simulink model "tqdtqr_rebuild_V3"  (R2021b)
settings: Solver=VariableStepAuto  StartTime=0.0  StopTime=10.0  RelTol=1e-3
undefined symbols (not defined in the file): ATQD_AfterTqMinGain_X_Deg, ATQD_APSCreepBaseTqD_X_kph, ATQD_APSCreepBaseTqD_Y_Deg, ATQD_APSCreepBaseTqR_X_kph, ATQD_APSCreepBaseTqR_Y_Deg, ATQD_APSCreepIterm_X_kph, ATQD_APSCreepIterm_Y_kph, ATQD_APSCreepPterm_X_kph, ATQD_APSCreepPterm_Y_kph, ATQD_APSDecReq_X_kph, ATQD_APSDecReq_Y_mps2, ATQD_APSDecReqCMD_X_kph, ATQD_APSDecReqTs_X_pct, ATQD_APSDecTimeGain_X_Deg, ATQD_APSDecTimeGain_Y_s, ATQD_APSReqLowSpd_X_Deg, ATQD_AutoHoldReleaseBPS_X_Deg, ATQD_AWDLoadTrqnsGain_X_kg, ATQD_AWDLoadTrqnsGain_Y_pct, ATQD_BOSEnBPSPosn_X_kph, ATQD_BOSMap_X_rpm, ATQD_BOSMap_Y_pct, ATQD_CreepBaseTqD_X_kph, ATQD_CreepBaseTqD_Y_Deg, ATQD_CreepBaseTqR_X_kph, ATQD_CreepBaseTqR_Y_Deg, ATQD_CreepBPSDisPosn_X_Deg, ATQD_CreepBPSDisPosnR_X_Deg, ATQD_CreepBPSEnPosn_X_Deg, ATQD_CreepBPSEnPosnR_X_Deg, ATQD_CreepDeltaTq_X_kph, ATQD_CreepIterm_X_kph, ATQD_CreepIterm_Y_kph, ATQD_CreepItermMaxLimit_X_pct, ATQD_CreepPreloadTime_X_kph, ATQD_CreepPreloadTq_X_kph, ATQD_CreepPreloadTq_Y_s, ATQD_CreepProtTq_X_Deg, ATQD_CreepPterm_X_kph, ATQD_CreepPterm_Y_kph, ATQD_CreepRrTqSpRat_X_rpm, ATQD_CreepRrTqSpRat_Y_Nm, ATQD_CreepTargetSpdD_X_pct, ATQD_CreepTargetSpdR_X_pct, ATQD_CreepUpLimitTq_X_rpm, ATQD_DecIneOPDHoldEnDelay_X_Deg, ATQD_DecIneOPDHoldEnDelay_Y_bar, ATQD_ECOTqMapD_X_rpm, ATQD_ECOTqMapD_Y_pct, ATQD_EMTqMapD_X_rpm, ATQD_EMTqMapD_Y_pct, ATQD_EOPDTqMapDCon_X_rpm, ATQD_EOPDTqMapDCon_Y_Deg, ATQD_EstInitVehWeight_X_c, ATQD_FAfterTqCMDGain_X_rpm, ATQD_FAfterTqCMDGain_Y_pct, ATQD_ForceLowSpd_X_Deg, ATQD_ForcePLimitSpd_X_Deg, ATQD_FrLossMAPLowV_X_rpm, ATQD_FrLossMAPLowV_Y_Nm ... (+949)
libraries: simulink x235, hcu_lib x208, tqr x63, tqd x6
(part 31 of 37)

== system tqdtqr_rebuild_V3/Input_Convert/Signal function/combo key/Combo Key Detection/DiagnosisOff Mode/Key1 ==
  VSCP_ComboKeyCMD_enum : Inport
  VSCP_ComboKeyEn_flg : Inport  Port=2
  VSCP_ComboKeyReset_flg : Inport  Port=3
  AND : Logic  Inputs=3  AllPortsSameDT=off  OutDataTypeStr=boolean
  Constant1 : Constant  Value=KTQD_DiagnosisOff1_enum
  Constant2 : Constant  Value=ENUM_COMBOKEY_NONE
  Constant4 : Constant  Value=ENUM_COMBOKEY_NONE
  Data Type Conversion : DataTypeConversion  OutDataTypeStr=uint8
  Delay : Delay  DelayLength=1  InitialCondition=uint8(0)
      settings: AttributesFormatString=%<InitialCondition>
  Delay1 : Delay  DelayLength=1  InitialCondition=uint8(0)
      settings: AttributesFormatString=%<InitialCondition>
  Detect Change : simulink/Logic and Bit Operations/Detect Change  vinit=boolean(0)  OutDataTypeStr=boolean
  Detect Increase : simulink/Logic and Bit Operations/Detect Increase  vinit=boolean(0)  OutDataTypeStr=boolean
  Equal : RelationalOperator  Operator===  OutDataTypeStr=boolean  RndMeth=Simplest
  Equal1 : RelationalOperator  Operator=~=  OutDataTypeStr=boolean  RndMeth=Simplest
  Equal2 : RelationalOperator  Operator===  OutDataTypeStr=boolean  RndMeth=Simplest
  If : If  NumInputs=2  IfExpression=u1 ~=0  ElseIfExpressions=u2 ~= 0
  Maintain : Subsystem  TreatAsAtomicUnit=on
  Merge : Merge  Inputs=3
  OR : Logic  Operator=OR  AllPortsSameDT=off  OutDataTypeStr=boolean
  Reset : Subsystem  TreatAsAtomicUnit=on
  Write : Subsystem  TreatAsAtomicUnit=on
  VSCP_ComboKey1_enum : Outport
  VSCP_Key1Pass_flg : Outport  Port=2
  wires:
  OR/1 -> [VSCP_ResetComboKey_flg]  "VSCP_ResetComboKey_flg"
  [VSCP_WriteComboCMD_flg] -> If/2
  [VSCP_ComboKeyCMD_enum] -> Equal1/1
  [VSCP_ComboKeyReset_flg] -> OR/2
  [VSCP_ComboKey1_enum] -> Delay/1
  Equal1/1 -> AND/2
  Constant2/1 -> Equal2/2
  Equal2/1 -> AND/3
  Reset/1(ResetToZero) -> Merge/1
  Merge/1 -> Data Type Conversion/1
  Delay/1 -> Equal2/1
  If/3 -> Maintain/Action
  Constant4/1 -> Equal1/2
  Maintain/1(KeepKey1) -> Merge/3
  Detect Change/1 -> AND/1
  [VSCP_ComboKeyEn_flg] -> Detect Increase/1
  [VSCP_ResetComboKey_flg] -> If/1
  [VSCP_ComboKeyCMD_enum] -> Detect Change/1
  [VSCP_ComboKeyCMD_enum] -> Write/1(Input)
  AND/1 -> [VSCP_WriteComboCMD_flg]  "VSCP_WriteComboCMD_flg"
  Detect Increase/1 -> OR/1
  If/1 -> Reset/Action
  Write/1(WriteCMD) -> Merge/2
  If/2 -> Write/Action
  [VSCP_ComboKey1_enum] -> Equal/1
  Constant1/1 -> Equal/2
  Equal/1 -> [VSCP_Key1Pass_flg]  "VTQD_DiagnosisOff1Pass_flg"
  VSCP_ComboKeyCMD_enum/1 -> [VSCP_ComboKeyCMD_enum]
  VSCP_ComboKeyReset_flg/1 -> [VSCP_ComboKeyReset_flg]
  VSCP_ComboKeyEn_flg/1 -> [VSCP_ComboKeyEn_flg]
  [VSCP_ComboKey1_enum] -> VSCP_ComboKey1_enum/1
  [VSCP_Key1Pass_flg] -> VSCP_Key1Pass_flg/1
  [VSCP_ComboKey1_enum] -> Delay1/1
  Delay1/1 -> Maintain/1(Input)
  Data Type Conversion/1 -> [VSCP_ComboKey1_enum]  "VTQD_DiagnosisOff1_enum"

== system tqdtqr_rebuild_V3/Input_Convert/Signal function/combo key/Combo Key Detection/DiagnosisOff Mode/Key2 ==
  VSCP_ComboKeyCMD_enum : Inport
  VSCP_ComboKeyEn_flg : Inport  Port=2
  VSCP_ComboKeyReset_flg : Inport  Port=3
  VSCP_ComboKey1_enum : Inport  Port=4
  AND : Logic  Inputs=4  AllPortsSameDT=off  OutDataTypeStr=boolean
  Constant1 : Constant  Value=KTQD_DiagnosisOff2_enum
  Constant2 : Constant  Value=ENUM_COMBOKEY_NONE
  Constant3 : Constant  Value=ENUM_COMBOKEY_NONE
  Constant4 : Constant  Value=ENUM_COMBOKEY_NONE  OutDataTypeStr=uint8
  Data Type Conversion : DataTypeConversion  OutDataTypeStr=uint8
  Delay : Delay  DelayLength=1  InitialCondition=uint8(0)
      settings: AttributesFormatString=%<InitialCondition>
  Delay1 : Delay  DelayLength=1  InitialCondition=uint8(0)
      settings: AttributesFormatString=%<InitialCondition>
  Delay2 : Delay  DelayLength=1  InitialCondition=uint8(0)
      settings: AttributesFormatString=%<InitialCondition>
  Detect Change : simulink/Logic and Bit Operations/Detect Change  vinit=boolean(0)  OutDataTypeStr=boolean
  Detect Increase : simulink/Logic and Bit Operations/Detect Increase  vinit=boolean(0)  OutDataTypeStr=boolean
  Equal : RelationalOperator  Operator===  OutDataTypeStr=boolean  RndMeth=Simplest
  Equal1 : RelationalOperator  Operator=~=  OutDataTypeStr=boolean  RndMeth=Simplest
  Equal2 : RelationalOperator  Operator=~=  OutDataTypeStr=boolean  RndMeth=Simplest
  Equal3 : RelationalOperator  Operator===  OutDataTypeStr=boolean  RndMeth=Simplest
  If : If  NumInputs=2  IfExpression=u1 ~=0  ElseIfExpressions=u2 ~= 0
  Maintain : Subsystem  TreatAsAtomicUnit=on
  Merge : Merge  Inputs=3
  OR : Logic  Operator=OR  AllPortsSameDT=off  OutDataTypeStr=boolean
  Reset : Subsystem  TreatAsAtomicUnit=on
  Write : Subsystem  TreatAsAtomicUnit=on
  VSCP_ComboKey2_enum : Outport
  VSCP_Key2Pass_flg : Outport  Port=2
  wires:
  [VSCP_Key2Pass_flg] -> VSCP_Key2Pass_flg/1
  [VSCP_ComboKey2_enum] -> VSCP_ComboKey2_enum/1
  VSCP_ComboKeyEn_flg/1 -> [VSCP_ComboKeyEn_flg]
  VSCP_ComboKeyReset_flg/1 -> [VSCP_ComboKeyReset_flg]
  VSCP_ComboKeyCMD_enum/1 -> [VSCP_ComboKeyCMD_enum]
  Equal/1 -> [VSCP_Key2Pass_flg]  "VTQD_DiagnosisOff2Pass_flg"
  Constant1/1 -> Equal/2
  [VSCP_ComboKey2_enum] -> Equal/1
  If/2 -> Write/Action
  Write/1(WriteCMD) -> Merge/2
  If/1 -> Reset/Action
  Detect Increase/1 -> OR/1
  AND/1 -> [VSCP_WriteComboCMD_flg]  "VSCP_WriteComboCMD_flg"
  [VSCP_ComboKeyCMD_enum] -> Write/1(Input)
  [VSCP_ComboKeyCMD_enum] -> Detect Change/1
  [VSCP_ResetComboKey_flg] -> If/1
  [VSCP_ComboKeyEn_flg] -> Detect Increase/1
  Detect Change/1 -> AND/1
  Maintain/1(KeepKey2) -> Merge/3
  Constant4/1 -> Equal1/2
  If/3 -> Maintain/Action
  Delay1/1 -> Equal2/1
  Merge/1 -> Data Type Conversion/1
  Reset/1(ResetToZero) -> Merge/1
  Equal2/1 -> AND/3
  Constant2/1 -> Equal2/2
  Equal1/1 -> AND/2
  [VSCP_ComboKey1_enum] -> Delay1/1
  [VSCP_ComboKeyReset_flg] -> OR/2
  [VSCP_ComboKeyCMD_enum] -> Equal1/1
  [VSCP_WriteComboCMD_flg] -> If/2
  OR/1 -> [VSCP_ResetComboKey_flg]  "VSCP_ResetComboKey_flg"
  VSCP_ComboKey1_enum/1 -> [VSCP_ComboKey1_enum]
  [VSCP_ComboKey2_enum] -> Delay/1
  Constant3/1 -> Equal3/2
  Delay/1 -> Equal3/1
  Equal3/1 -> AND/4
  Delay2/1 -> Maintain/1(Input)
  [VSCP_ComboKey2_enum] -> Delay2/1
  Data Type Conversion/1 -> [VSCP_ComboKey2_enum]  "VTQD_DiagnosisOff2_enum"

== system tqdtqr_rebuild_V3/Input_Convert/Signal function/combo key/Combo Key Detection/DiagnosisOff Mode/Key3 ==
  VSCP_ComboKeyCMD_enum : Inport
  VSCP_ComboKeyEn_flg : Inport  Port=2
  VSCP_ComboKeyReset_flg : Inport  Port=3
  VSCP_ComboKey2_enum : Inport  Port=4
  AND : Logic  Inputs=4  AllPortsSameDT=off  OutDataTypeStr=boolean
  Constant1 : Constant  Value=KTQD_DiagnosisOff3_enum
  Constant2 : Constant  Value=ENUM_COMBOKEY_NONE
  Constant3 : Constant  Value=ENUM_COMBOKEY_NONE
  Constant4 : Constant  Value=ENUM_COMBOKEY_NONE
  Data Type Conversion : DataTypeConversion  OutDataTypeStr=uint8
  Delay : Delay  DelayLength=1  InitialCondition=uint8(0)
      settings: AttributesFormatString=%<InitialCondition>
  Delay1 : Delay  DelayLength=1  InitialCondition=uint8(0)
      settings: AttributesFormatString=%<InitialCondition>
  Delay2 : Delay  DelayLength=1  InitialCondition=uint8(0)
      settings: AttributesFormatString=%<InitialCondition>
  Detect Change : simulink/Logic and Bit Operations/Detect Change  vinit=boolean(0)  OutDataTypeStr=boolean
  Detect Increase : simulink/Logic and Bit Operations/Detect Increase  vinit=boolean(0)  OutDataTypeStr=boolean
  Equal : RelationalOperator  Operator===  OutDataTypeStr=boolean  RndMeth=Simplest
  Equal1 : RelationalOperator  Operator=~=  OutDataTypeStr=boolean  RndMeth=Simplest
  Equal2 : RelationalOperator  Operator=~=  OutDataTypeStr=boolean  RndMeth=Simplest
  Equal3 : RelationalOperator  Operator===  OutDataTypeStr=boolean  RndMeth=Simplest
  If : If  NumInputs=2  IfExpression=u1 ~=0  ElseIfExpressions=u2 ~= 0
  Maintain : Subsystem  TreatAsAtomicUnit=on
  Merge : Merge  Inputs=3
  OR : Logic  Operator=OR  AllPortsSameDT=off  OutDataTypeStr=boolean
  Reset : Subsystem  TreatAsAtomicUnit=on
  Write : Subsystem  TreatAsAtomicUnit=on
  VSCP_ComboKey3_enum : Outport
  VSCP_Key3Pass_flg : Outport  Port=2
  wires:
  VSCP_ComboKey2_enum/1 -> [VSCP_ComboKey2_enum]
  OR/1 -> [VSCP_ResetComboKey_flg]  "VSCP_ResetComboKey_flg"
  [VSCP_WriteComboCMD_flg] -> If/2
  [VSCP_ComboKeyCMD_enum] -> Equal1/1
  [VSCP_ComboKeyReset_flg] -> OR/2
  [VSCP_ComboKey2_enum] -> Delay1/1
  Equal1/1 -> AND/2
  Constant2/1 -> Equal2/2
  Equal2/1 -> AND/3
  Reset/1(ResetToZero) -> Merge/1
  Merge/1 -> Data Type Conversion/1
  Delay1/1 -> Equal2/1
  If/3 -> Maintain/Action
  Constant4/1 -> Equal1/2
  Maintain/1(KeepKey3) -> Merge/3
  Detect Change/1 -> AND/1
  [VSCP_ComboKeyEn_flg] -> Detect Increase/1
  [VSCP_ResetComboKey_flg] -> If/1
  [VSCP_ComboKeyCMD_enum] -> Detect Change/1
  [VSCP_ComboKeyCMD_enum] -> Write/1(Input)
  AND/1 -> [VSCP_WriteComboCMD_flg]  "VSCP_WriteComboCMD_flg"
  Detect Increase/1 -> OR/1
  If/1 -> Reset/Action
  Write/1(WriteCMD) -> Merge/2
  If/2 -> Write/Action
  Constant1/1 -> Equal/2
  Equal/1 -> [VSCP_Key3Pass_flg]  "VTQD_DiagnosisOff3Pass_flg"
  VSCP_ComboKeyCMD_enum/1 -> [VSCP_ComboKeyCMD_enum]
  VSCP_ComboKeyReset_flg/1 -> [VSCP_ComboKeyReset_flg]
  VSCP_ComboKeyEn_flg/1 -> [VSCP_ComboKeyEn_flg]
  [VSCP_ComboKey3_enum] -> VSCP_ComboKey3_enum/1
  [VSCP_ComboKey3_enum] -> Equal/1
  [VSCP_Key3Pass_flg] -> VSCP_Key3Pass_flg/1
  Delay/1 -> Equal3/1
  Equal3/1 -> AND/4
  Constant3/1 -> Equal3/2
  [VSCP_ComboKey3_enum] -> Delay/1
  Delay2/1 -> Maintain/1(Input)
  [VSCP_ComboKey3_enum] -> Delay2/1
  Data Type Conversion/1 -> [VSCP_ComboKey3_enum]  "VTQD_DiagnosisOff3_enum"

== system tqdtqr_rebuild_V3/Input_Convert/Signal function/combo key/Combo Key Detection/DiagnosisOff Mode/Key4 ==
  VSCP_ComboKeyCMD_enum : Inport
  VSCP_ComboKeyEn_flg : Inport  Port=2
  VSCP_ComboKeyReset_flg : Inport  Port=3
  VSCP_ComboKey3_enum : Inport  Port=4
  AND : Logic  Inputs=4  AllPortsSameDT=off  OutDataTypeStr=boolean
  Constant1 : Constant  Value=KTQD_DiagnosisOff4_enum
  Constant2 : Constant  Value=ENUM_COMBOKEY_NONE
  Constant3 : Constant  Value=ENUM_COMBOKEY_NONE
  Constant4 : Constant  Value=ENUM_COMBOKEY_NONE
  Data Type Conversion : DataTypeConversion  OutDataTypeStr=uint8
  Delay : Delay  DelayLength=1  InitialCondition=uint8(0)
      settings: AttributesFormatString=%<InitialCondition>
  Delay1 : Delay  DelayLength=1  InitialCondition=uint8(0)
      settings: AttributesFormatString=%<InitialCondition>
  Delay2 : Delay  DelayLength=1  InitialCondition=uint8(0)
      settings: AttributesFormatString=%<InitialCondition>
  Detect Change : simulink/Logic and Bit Operations/Detect Change  vinit=boolean(0)  OutDataTypeStr=boolean
  Detect Increase : simulink/Logic and Bit Operations/Detect Increase  vinit=boolean(0)  OutDataTypeStr=boolean
  Equal : RelationalOperator  Operator===  OutDataTypeStr=boolean  RndMeth=Simplest
  Equal1 : RelationalOperator  Operator=~=  OutDataTypeStr=boolean  RndMeth=Simplest
  Equal2 : RelationalOperator  Operator=~=  OutDataTypeStr=boolean  RndMeth=Simplest
  Equal3 : RelationalOperator  Operator===  OutDataTypeStr=boolean  RndMeth=Simplest
  If : If  NumInputs=2  IfExpression=u1 ~=0  ElseIfExpressions=u2 ~= 0
  Maintain : Subsystem  TreatAsAtomicUnit=on
  Merge : Merge  Inputs=3
  OR : Logic  Operator=OR  AllPortsSameDT=off  OutDataTypeStr=boolean
  Reset : Subsystem  TreatAsAtomicUnit=on
  Write : Subsystem  TreatAsAtomicUnit=on
  VSCP_ComboKey4_enum : Outport
  VSCP_Key4Pass_flg : Outport  Port=2
  wires:
  [VSCP_ComboKey4_enum] -> Equal/1
  VSCP_ComboKeyEn_flg/1 -> [VSCP_ComboKeyEn_flg]
  VSCP_ComboKeyReset_flg/1 -> [VSCP_ComboKeyReset_flg]
  VSCP_ComboKeyCMD_enum/1 -> [VSCP_ComboKeyCMD_enum]
  Equal/1 -> [VSCP_Key4Pass_flg]  "VTQD_DiagnosisOff4Pass_flg"
  Constant1/1 -> Equal/2
  If/2 -> Write/Action
  Write/1(WriteCMD) -> Merge/2
  If/1 -> Reset/Action
  Detect Increase/1 -> OR/1
  AND/1 -> [VSCP_WriteComboCMD_flg]  "VSCP_WriteComboCMD_flg"
  [VSCP_ComboKeyCMD_enum] -> Write/1(Input)
  [VSCP_ComboKeyCMD_enum] -> Detect Change/1
  [VSCP_ResetComboKey_flg] -> If/1
  [VSCP_ComboKeyEn_flg] -> Detect Increase/1
  Detect Change/1 -> AND/1
  Maintain/1(KeepKey4) -> Merge/3
  Constant4/1 -> Equal1/2
  If/3 -> Maintain/Action
  Delay1/1 -> Equal2/1
  Merge/1 -> Data Type Conversion/1
  Reset/1(ResetToZero) -> Merge/1
  Equal2/1 -> AND/3
  Constant2/1 -> Equal2/2
  Equal1/1 -> AND/2
  [VSCP_ComboKey3_enum] -> Delay1/1
  [VSCP_ComboKeyReset_flg] -> OR/2
  [VSCP_ComboKeyCMD_enum] -> Equal1/1
  [VSCP_WriteComboCMD_flg] -> If/2
  OR/1 -> [VSCP_ResetComboKey_flg]  "VSCP_ResetComboKey_flg"
  VSCP_ComboKey3_enum/1 -> [VSCP_ComboKey3_enum]
  [VSCP_ComboKey4_enum] -> Delay/1
  Constant3/1 -> Equal3/2
  Delay/1 -> Equal3/1
  Equal3/1 -> AND/4
  [VSCP_Key4Pass_flg] -> VSCP_Key4Pass_flg/1
  [VSCP_ComboKey4_enum] -> VSCP_ComboKey4_enum/1
  [VSCP_ComboKey4_enum] -> Delay2/1
  Delay2/1 -> Maintain/1(Input)
  Data Type Conversion/1 -> [VSCP_ComboKey4_enum]  "VTQD_DiagnosisOff4_enum"

== system tqdtqr_rebuild_V3/Input_Convert/Signal function/combo key/Combo Key Detection/DiagnosisOff Mode/Key5 ==
  VSCP_ComboKeyCMD_enum : Inport
  VSCP_ComboKeyEn_flg : Inport  Port=2
  VSCP_ComboKeyReset_flg : Inport  Port=3
  VSCP_ComboKey4_enum : Inport  Port=4
  AND : Logic  Inputs=4  AllPortsSameDT=off  OutDataTypeStr=boolean
  Constant1 : Constant  Value=KTQD_DiagnosisOff5_enum
  Constant2 : Constant  Value=ENUM_COMBOKEY_NONE
  Constant3 : Constant  Value=ENUM_COMBOKEY_NONE
  Constant4 : Constant  Value=ENUM_COMBOKEY_NONE
  Data Type Conversion : DataTypeConversion  OutDataTypeStr=uint8
  Delay : Delay  DelayLength=1  InitialCondition=uint8(0)
      settings: AttributesFormatString=%<InitialCondition>
  Delay1 : Delay  DelayLength=1  InitialCondition=uint8(0)
      settings: AttributesFormatString=%<InitialCondition>
  Delay2 : Delay  DelayLength=1  InitialCondition=uint8(0)
      settings: AttributesFormatString=%<InitialCondition>
  Detect Change : simulink/Logic and Bit Operations/Detect Change  vinit=boolean(0)  OutDataTypeStr=boolean
  Detect Increase : simulink/Logic and Bit Operations/Detect Increase  vinit=boolean(0)  OutDataTypeStr=boolean
  Equal : RelationalOperator  Operator===  OutDataTypeStr=boolean  RndMeth=Simplest
  Equal1 : RelationalOperator  Operator=~=  OutDataTypeStr=boolean  RndMeth=Simplest
  Equal2 : RelationalOperator  Operator=~=  OutDataTypeStr=boolean  RndMeth=Simplest
  Equal3 : RelationalOperator  Operator===  OutDataTypeStr=boolean  RndMeth=Simplest
  If : If  NumInputs=2  IfExpression=u1 ~=0  ElseIfExpressions=u2 ~= 0
  Maintain : Subsystem  TreatAsAtomicUnit=on
  Merge : Merge  Inputs=3
  OR : Logic  Operator=OR  AllPortsSameDT=off  OutDataTypeStr=boolean
  Reset : Subsystem  TreatAsAtomicUnit=on
  Write : Subsystem  TreatAsAtomicUnit=on
  VSCP_ComboKey5_enum : Outport
  VSCP_Key5Pass_flg : Outport  Port=2
  wires:
  [VSCP_Key5Pass_flg] -> VSCP_Key5Pass_flg/1
  Equal3/1 -> AND/4
  Delay1/1 -> Equal3/1
  Constant3/1 -> Equal3/2
  [VSCP_ComboKey5_enum] -> Delay1/1
  VSCP_ComboKey4_enum/1 -> [VSCP_ComboKey4_enum]
  OR/1 -> [VSCP_ResetComboKey_flg]  "VSCP_ResetComboKey_flg"
  [VSCP_WriteComboCMD_flg] -> If/2
  [VSCP_ComboKeyCMD_enum] -> Equal1/1
  [VSCP_ComboKeyReset_flg] -> OR/2
  [VSCP_ComboKey4_enum] -> Delay/1
  Equal1/1 -> AND/2
  Constant2/1 -> Equal2/2
  Equal2/1 -> AND/3
  Reset/1(ResetToZero) -> Merge/1
  Merge/1 -> Data Type Conversion/1
  Delay/1 -> Equal2/1
  If/3 -> Maintain/Action
  Constant4/1 -> Equal1/2
  Maintain/1(KeepKey5) -> Merge/3
  Detect Change/1 -> AND/1
  [VSCP_ComboKeyEn_flg] -> Detect Increase/1
  [VSCP_ResetComboKey_flg] -> If/1
  [VSCP_ComboKeyCMD_enum] -> Detect Change/1
  [VSCP_ComboKeyCMD_enum] -> Write/1(Input)
  AND/1 -> [VSCP_WriteComboCMD_flg]  "VSCP_WriteComboCMD_flg"
  Detect Increase/1 -> OR/1
  If/1 -> Reset/Action
  Write/1(WriteCMD) -> Merge/2
  If/2 -> Write/Action
  Constant1/1 -> Equal/2
  Equal/1 -> [VSCP_Key5Pass_flg]  "VTQD_DiagnosisOff5Pass_flg"
  VSCP_ComboKeyCMD_enum/1 -> [VSCP_ComboKeyCMD_enum]
  VSCP_ComboKeyReset_flg/1 -> [VSCP_ComboKeyReset_flg]
  VSCP_ComboKeyEn_flg/1 -> [VSCP_ComboKeyEn_flg]
  [VSCP_ComboKey5_enum] -> Equal/1
  [VSCP_ComboKey5_enum] -> VSCP_ComboKey5_enum/1
  [VSCP_ComboKey5_enum] -> Delay2/1
  Delay2/1 -> Maintain/1(Input)
  Data Type Conversion/1 -> [VSCP_ComboKey5_enum]  "VTQD_DiagnosisOff5_enum"

== system tqdtqr_rebuild_V3/Input_Convert/Signal function/combo key/Combo Key Detection/DiagnosisOff Mode/Key6 ==
  VSCP_ComboKeyCMD_enum : Inport
  VSCP_ComboKeyEn_flg : Inport  Port=2
  VSCP_ComboKeyReset_flg : Inport  Port=3
  VSCP_ComboKey5_enum : Inport  Port=4
  AND : Logic  Inputs=4  AllPortsSameDT=off  OutDataTypeStr=boolean
  Constant1 : Constant  Value=KTQD_DiagnosisOff6_enum
  Constant2 : Constant  Value=ENUM_COMBOKEY_NONE
  Constant3 : Constant  Value=ENUM_COMBOKEY_NONE
  Constant4 : Constant  Value=ENUM_COMBOKEY_NONE
  Data Type Conversion : DataTypeConversion  OutDataTypeStr=uint8
  Delay : Delay  DelayLength=1  InitialCondition=uint8(0)
      settings: AttributesFormatString=%<InitialCondition>
  Delay1 : Delay  DelayLength=1  InitialCondition=uint8(0)
      settings: AttributesFormatString=%<InitialCondition>
  Delay3 : Delay  DelayLength=1  InitialCondition=uint8(0)
      settings: AttributesFormatString=%<InitialCondition>
  Detect Change : simulink/Logic and Bit Operations/Detect Change  vinit=boolean(0)  OutDataTypeStr=boolean
  Detect Increase : simulink/Logic and Bit Operations/Detect Increase  vinit=boolean(0)  OutDataTypeStr=boolean
  Equal : RelationalOperator  Operator===  OutDataTypeStr=boolean  RndMeth=Simplest
  Equal1 : RelationalOperator  Operator=~=  OutDataTypeStr=boolean  RndMeth=Simplest
  Equal2 : RelationalOperator  Operator=~=  OutDataTypeStr=boolean  RndMeth=Simplest
  Equal3 : RelationalOperator  Operator===  OutDataTypeStr=boolean  RndMeth=Simplest
  If : If  NumInputs=2  IfExpression=u1 ~=0  ElseIfExpressions=u2 ~= 0
  Maintain : Subsystem  TreatAsAtomicUnit=on
  Merge : Merge  Inputs=3
  OR : Logic  Operator=OR  AllPortsSameDT=off  OutDataTypeStr=boolean
  Reset : Subsystem  TreatAsAtomicUnit=on
  Write : Subsystem  TreatAsAtomicUnit=on
  VSCP_ComboKey6_enum : Outport
  VSCP_Key6Pass_flg : Outport  Port=2
  wires:
  [VSCP_ComboKey6_enum] -> VSCP_ComboKey6_enum/1
  [VSCP_ComboKey6_enum] -> Equal/1
  VSCP_ComboKeyEn_flg/1 -> [VSCP_ComboKeyEn_flg]
  VSCP_ComboKeyReset_flg/1 -> [VSCP_ComboKeyReset_flg]
  VSCP_ComboKeyCMD_enum/1 -> [VSCP_ComboKeyCMD_enum]
  Equal/1 -> [VSCP_Key6Pass_flg]  "VTQD_DiagnosisOff6Pass_flg"
  Constant1/1 -> Equal/2
  If/2 -> Write/Action
  Write/1(WriteCMD) -> Merge/2
  If/1 -> Reset/Action
  Detect Increase/1 -> OR/1
  AND/1 -> [VSCP_WriteComboCMD_flg]  "VSCP_WriteComboCMD_flg"
  [VSCP_ComboKeyCMD_enum] -> Write/1(Input)
  [VSCP_ComboKeyCMD_enum] -> Detect Change/1
  [VSCP_ResetComboKey_flg] -> If/1
  [VSCP_ComboKeyEn_flg] -> Detect Increase/1
  Detect Change/1 -> AND/1
  Maintain/1(KeepKey6) -> Merge/3
  Constant4/1 -> Equal1/2
  If/3 -> Maintain/Action
  Delay1/1 -> Equal2/1
  Merge/1 -> Data Type Conversion/1
  Reset/1(ResetToZero) -> Merge/1
  Equal2/1 -> AND/3
  Constant2/1 -> Equal2/2
  Equal1/1 -> AND/2
  [VSCP_ComboKey5_enum] -> Delay1/1
  [VSCP_ComboKeyReset_flg] -> OR/2
  [VSCP_ComboKeyCMD_enum] -> Equal1/1
  [VSCP_WriteComboCMD_flg] -> If/2
  OR/1 -> [VSCP_ResetComboKey_flg]  "VSCP_ResetComboKey_flg"
  VSCP_ComboKey5_enum/1 -> [VSCP_ComboKey5_enum]
  [VSCP_ComboKey6_enum] -> Delay/1
  Constant3/1 -> Equal3/2
  Delay/1 -> Equal3/1
  Equal3/1 -> AND/4
  [VSCP_Key6Pass_flg] -> VSCP_Key6Pass_flg/1
  Delay3/1 -> Maintain/1(Input)
  [VSCP_ComboKey6_enum] -> Delay3/1
  Data Type Conversion/1 -> [VSCP_ComboKey6_enum]  "VTQD_DiagnosisOff6_enum"

== system tqdtqr_rebuild_V3/Input_Convert/Signal function/combo key/Combo Key Detection/DiagnosisOff Mode/Key7 ==
  VSCP_ComboKeyCMD_enum : Inport
  VSCP_ComboKeyEn_flg : Inport  Port=2
  VSCP_ComboKeyReset_flg : Inport  Port=3
  VSCP_ComboKey6_enum : Inport  Port=4
  AND : Logic  Inputs=4  AllPortsSameDT=off  OutDataTypeStr=boolean
  Constant1 : Constant  Value=KTQD_DiagnosisOff7_enum
  Constant2 : Constant  Value=ENUM_COMBOKEY_NONE  OutDataTypeStr=uint8
  Constant3 : Constant  Value=ENUM_COMBOKEY_NONE
  Constant4 : Constant  Value=ENUM_COMBOKEY_NONE  OutDataTypeStr=uint8
  Data Type Conversion : DataTypeConversion  OutDataTypeStr=uint8
  Delay1 : Delay  DelayLength=1  InitialCondition=uint8(0)
      settings: AttributesFormatString=%<InitialCondition>
  Delay2 : Delay  DelayLength=1  InitialCondition=uint8(0)
      settings: AttributesFormatString=%<InitialCondition>
  Delay3 : Delay  DelayLength=1  InitialCondition=uint8(0)
      settings: AttributesFormatString=%<InitialCondition>
  Detect Change : simulink/Logic and Bit Operations/Detect Change  vinit=boolean(0)  OutDataTypeStr=boolean
  Detect Increase : simulink/Logic and Bit Operations/Detect Increase  vinit=boolean(0)  OutDataTypeStr=boolean
  Equal : RelationalOperator  Operator===  OutDataTypeStr=boolean  RndMeth=Simplest
  Equal1 : RelationalOperator  Operator=~=  OutDataTypeStr=boolean  RndMeth=Simplest
  Equal2 : RelationalOperator  Operator=~=  OutDataTypeStr=boolean  RndMeth=Simplest
  Equal3 : RelationalOperator  Operator===  OutDataTypeStr=boolean  RndMeth=Simplest
  If : If  NumInputs=2  IfExpression=u1 ~=0  ElseIfExpressions=u2 ~= 0
  Maintain : Subsystem  TreatAsAtomicUnit=on
  Merge : Merge  Inputs=3
  OR : Logic  Operator=OR  AllPortsSameDT=off  OutDataTypeStr=boolean
  Reset : Subsystem  TreatAsAtomicUnit=on
  Write : Subsystem  TreatAsAtomicUnit=on
  VSCP_ComboKey7_enum : Outport
  VSCP_Key7Pass_flg : Outport  Port=2
  wires:
  [VSCP_Key7Pass_flg] -> VSCP_Key7Pass_flg/1
  Equal3/1 -> AND/4
  Delay3/1 -> Equal3/1
  Constant3/1 -> Equal3/2
  [VSCP_ComboKey7_enum] -> Delay3/1
  VSCP_ComboKey6_enum/1 -> [VSCP_ComboKey6_enum]
  OR/1 -> [VSCP_ResetComboKey_flg]  "VSCP_ResetComboKey_flg"
  [VSCP_WriteComboCMD_flg] -> If/2
  [VSCP_ComboKeyCMD_enum] -> Equal1/1
  [VSCP_ComboKeyReset_flg] -> OR/2
  [VSCP_ComboKey6_enum] -> Delay1/1
  Equal1/1 -> AND/2
  Constant2/1 -> Equal2/2
  Equal2/1 -> AND/3
  Reset/1(ResetToZero) -> Merge/1
  Merge/1 -> Data Type Conversion/1
  Delay1/1 -> Equal2/1
  If/3 -> Maintain/Action
  Constant4/1 -> Equal1/2
  Maintain/1(KeepKey7) -> Merge/3
  Detect Change/1 -> AND/1
  [VSCP_ComboKeyEn_flg] -> Detect Increase/1
  [VSCP_ResetComboKey_flg] -> If/1
  [VSCP_ComboKeyCMD_enum] -> Detect Change/1
  [VSCP_ComboKeyCMD_enum] -> Write/1(Input)
  AND/1 -> [VSCP_WriteComboCMD_flg]  "VSCP_WriteComboCMD_flg"
  Detect Increase/1 -> OR/1
  If/1 -> Reset/Action
  Write/1(WriteCMD) -> Merge/2
  If/2 -> Write/Action
  Constant1/1 -> Equal/2
  Equal/1 -> [VSCP_Key7Pass_flg]  "VTQD_DiagnosisOff7Pass_flg"
  VSCP_ComboKeyCMD_enum/1 -> [VSCP_ComboKeyCMD_enum]
  VSCP_ComboKeyReset_flg/1 -> [VSCP_ComboKeyReset_flg]
  VSCP_ComboKeyEn_flg/1 -> [VSCP_ComboKeyEn_flg]
  [VSCP_ComboKey7_enum] -> Equal/1
  [VSCP_ComboKey7_enum] -> VSCP_ComboKey7_enum/1
  [VSCP_ComboKey7_enum] -> Delay2/1
  Delay2/1 -> Maintain/1(Input)
  Data Type Conversion/1 -> [VSCP_ComboKey7_enum]  "VTQD_DiagnosisOff7_enum"

== system tqdtqr_rebuild_V3/Input_Convert/Signal function/combo key/Combo Key Detection/DiagnosisOff Mode/Key8 ==
  VSCP_ComboKeyCMD_enum : Inport
  VSCP_ComboKeyEn_flg : Inport  Port=2
  VSCP_ComboKeyReset_flg : Inport  Port=3
  VSCP_ComboKey7_enum : Inport  Port=4
  AND : Logic  Inputs=4  AllPortsSameDT=off  OutDataTypeStr=boolean
  Constant1 : Constant  Value=KTQD_DiagnosisOff8_enum
  Constant2 : Constant  Value=ENUM_COMBOKEY_NONE
  Constant3 : Constant  Value=ENUM_COMBOKEY_NONE
  Constant4 : Constant  Value=ENUM_COMBOKEY_NONE
  Data Type Conversion : DataTypeConversion  OutDataTypeStr=uint8
  Delay1 : Delay  DelayLength=1  InitialCondition=uint8(0)
      settings: AttributesFormatString=%<InitialCondition>
  Delay2 : Delay  DelayLength=1  InitialCondition=uint8(0)
      settings: AttributesFormatString=%<InitialCondition>
  Delay3 : Delay  DelayLength=1  InitialCondition=uint8(0)
      settings: AttributesFormatString=%<InitialCondition>
  Detect Change : simulink/Logic and Bit Operations/Detect Change  vinit=boolean(0)  OutDataTypeStr=boolean
  Detect Increase : simulink/Logic and Bit Operations/Detect Increase  vinit=boolean(0)  OutDataTypeStr=boolean
  Equal : RelationalOperator  Operator===  OutDataTypeStr=boolean  RndMeth=Simplest
  Equal1 : RelationalOperator  Operator=~=  OutDataTypeStr=boolean  RndMeth=Simplest
  Equal2 : RelationalOperator  Operator=~=  OutDataTypeStr=boolean  RndMeth=Simplest
  Equal3 : RelationalOperator  Operator===  OutDataTypeStr=boolean  RndMeth=Simplest
  If : If  NumInputs=2  IfExpression=u1 ~=0  ElseIfExpressions=u2 ~= 0
  Maintain : Subsystem  TreatAsAtomicUnit=on
  Merge : Merge  Inputs=3
  OR : Logic  Operator=OR  AllPortsSameDT=off  OutDataTypeStr=boolean
  Reset : Subsystem  TreatAsAtomicUnit=on
  Write : Subsystem  TreatAsAtomicUnit=on
  VSCP_ComboKey8_enum : Outport
  VSCP_Key8Pass_flg : Outport  Port=2
  wires:
  VSCP_ComboKeyEn_flg/1 -> [VSCP_ComboKeyEn_flg]
  VSCP_ComboKeyReset_flg/1 -> [VSCP_ComboKeyReset_flg]
  VSCP_ComboKeyCMD_enum/1 -> [VSCP_ComboKeyCMD_enum]
  Equal/1 -> [VSCP_Key8Pass_flg]  "VTQD_DiagnosisOff8Pass_flg"
  Constant1/1 -> Equal/2
  If/2 -> Write/Action
  Write/1(WriteCMD) -> Merge/2
  If/1 -> Reset/Action
  Detect Increase/1 -> OR/1
  AND/1 -> [VSCP_WriteComboCMD_flg]  "VSCP_WriteComboCMD_flg"
  [VSCP_ComboKeyCMD_enum] -> Write/1(Input)
  [VSCP_ComboKeyCMD_enum] -> Detect Change/1
  [VSCP_ResetComboKey_flg] -> If/1
  [VSCP_ComboKeyEn_flg] -> Detect Increase/1
  Detect Change/1 -> AND/1
  Maintain/1(KeepKey8) -> Merge/3
  Constant4/1 -> Equal1/2
  If/3 -> Maintain/Action
  Delay3/1 -> Equal2/1
  Merge/1 -> Data Type Conversion/1
  Reset/1(ResetToZero) -> Merge/1
  Equal2/1 -> AND/3
  Constant2/1 -> Equal2/2
  Equal1/1 -> AND/2
  [VSCP_ComboKey7_enum] -> Delay3/1
  [VSCP_ComboKeyReset_flg] -> OR/2
  [VSCP_ComboKeyCMD_enum] -> Equal1/1
  [VSCP_WriteComboCMD_flg] -> If/2
  OR/1 -> [VSCP_ResetComboKey_flg]  "VSCP_ResetComboKey_flg"
  VSCP_ComboKey7_enum/1 -> [VSCP_ComboKey7_enum]
  [VSCP_ComboKey8_enum] -> Delay1/1
  Constant3/1 -> Equal3/2
  Delay1/1 -> Equal3/1
  Equal3/1 -> AND/4
  [VSCP_Key8Pass_flg] -> VSCP_Key8Pass_flg/1
  [VSCP_ComboKey8_enum] -> Equal/1
  [VSCP_ComboKey8_enum] -> VSCP_ComboKey8_enum/1
  [VSCP_ComboKey8_enum] -> Delay2/1
  Delay2/1 -> Maintain/1(Input)
  Data Type Conversion/1 -> [VSCP_ComboKey8_enum]  "VTQD_DiagnosisOff8_enum"

== system tqdtqr_rebuild_V3/Input_Convert/Signal function/combo key/Combo Key Detection/Engineering Mode/Key1 ==
  VSCP_ComboKeyCMD_enum : Inport
  VSCP_ComboKeyEn_flg : Inport  Port=2
  VSCP_ComboKeyReset_flg : Inport  Port=3
  AND : Logic  Inputs=3  AllPortsSameDT=off  OutDataTypeStr=boolean
  Constant1 : Constant  Value=KTQD_Engineering1_enum
  Constant2 : Constant  Value=ENUM_COMBOKEY_NONE
  Constant4 : Constant  Value=ENUM_COMBOKEY_NONE
  Data Type Conversion : DataTypeConversion  OutDataTypeStr=uint8
  Delay : Delay  DelayLength=1  InitialCondition=uint8(0)
      settings: AttributesFormatString=%<InitialCondition>
  Delay1 : Delay  DelayLength=1  InitialCondition=uint8(0)
      settings: AttributesFormatString=%<InitialCondition>
  Detect Change : simulink/Logic and Bit Operations/Detect Change  vinit=boolean(0)  OutDataTypeStr=boolean
  Detect Change1 : simulink/Logic and Bit Operations/Detect Change  vinit=boolean(0)  OutDataTypeStr=boolean
  Equal : RelationalOperator  Operator===  OutDataTypeStr=boolean  RndMeth=Simplest
  Equal1 : RelationalOperator  Operator=~=  OutDataTypeStr=boolean  RndMeth=Simplest
  Equal2 : RelationalOperator  Operator===  OutDataTypeStr=boolean  RndMeth=Simplest
  If : If  NumInputs=2  IfExpression=u1 ~=0  ElseIfExpressions=u2 ~= 0
  Maintain : Subsystem  TreatAsAtomicUnit=on
  Merge : Merge  Inputs=3
  OR : Logic  Operator=OR  AllPortsSameDT=off  OutDataTypeStr=boolean
  Reset : Subsystem  TreatAsAtomicUnit=on
  Write : Subsystem  TreatAsAtomicUnit=on
  VSCP_ComboKey1_enum : Outport
  VSCP_Key1Pass_flg : Outport  Port=2
  wires:
  Data Type Conversion/1 -> [VSCP_ComboKey1_enum]  "VTQD_Engineering1_enum"
  Delay1/1 -> Maintain/1(Input)
  [VSCP_ComboKey1_enum] -> Delay1/1
  [VSCP_Key1Pass_flg] -> VSCP_Key1Pass_flg/1
  [VSCP_ComboKey1_enum] -> VSCP_ComboKey1_enum/1
  VSCP_ComboKeyEn_flg/1 -> [VSCP_ComboKeyEn_flg]
  VSCP_ComboKeyReset_flg/1 -> [VSCP_ComboKeyReset_flg]
  VSCP_ComboKeyCMD_enum/1 -> [VSCP_ComboKeyCMD_enum]
  Equal/1 -> [VSCP_Key1Pass_flg]  "VTQD_Engineering1Pass_flg"
  Constant1/1 -> Equal/2
  [VSCP_ComboKey1_enum] -> Equal/1
  If/2 -> Write/Action
  Write/1(WriteCMD) -> Merge/2
  If/1 -> Reset/Action
  Detect Change1/1 -> OR/1
  AND/1 -> [VSCP_WriteComboCMD_flg]  "VSCP_WriteComboCMD_flg"
  [VSCP_ComboKeyCMD_enum] -> Write/1(Input)
  [VSCP_ComboKeyCMD_enum] -> Detect Change/1
  [VSCP_ResetComboKey_flg] -> If/1
  [VSCP_ComboKeyEn_flg] -> Detect Change1/1
  Detect Change/1 -> AND/1
  Maintain/1(KeepKey1) -> Merge/3
  Constant4/1 -> Equal1/2
  If/3 -> Maintain/Action
  Delay/1 -> Equal2/1
  Merge/1 -> Data Type Conversion/1
  Reset/1(ResetToZero) -> Merge/1
  Equal2/1 -> AND/3
  Constant2/1 -> Equal2/2
  Equal1/1 -> AND/2
  [VSCP_ComboKey1_enum] -> Delay/1
  [VSCP_ComboKeyReset_flg] -> OR/2
  [VSCP_ComboKeyCMD_enum] -> Equal1/1
  [VSCP_WriteComboCMD_flg] -> If/2
  OR/1 -> [VSCP_ResetComboKey_flg]  "VSCP_ResetComboKey_flg"

== system tqdtqr_rebuild_V3/Input_Convert/Signal function/combo key/Combo Key Detection/Engineering Mode/Key2 ==
  VSCP_ComboKeyCMD_enum : Inport
  VSCP_ComboKeyEn_flg : Inport  Port=2
  VSCP_ComboKeyReset_flg : Inport  Port=3
  VSCP_ComboKey1_enum : Inport  Port=4
  AND : Logic  Inputs=4  AllPortsSameDT=off  OutDataTypeStr=boolean
  Constant1 : Constant  Value=KTQD_Engineering2_enum
  Constant2 : Constant  Value=ENUM_COMBOKEY_NONE
  Constant3 : Constant  Value=ENUM_COMBOKEY_NONE
  Constant4 : Constant  Value=ENUM_COMBOKEY_NONE  OutDataTypeStr=uint8
  Data Type Conversion : DataTypeConversion  OutDataTypeStr=uint8
  Delay : Delay  DelayLength=1  InitialCondition=uint8(0)
      settings: AttributesFormatString=%<InitialCondition>
  Delay1 : Delay  DelayLength=1  InitialCondition=uint8(0)
      settings: AttributesFormatString=%<InitialCondition>
  Delay2 : Delay  DelayLength=1  InitialCondition=uint8(0)
      settings: AttributesFormatString=%<InitialCondition>
  Detect Change : simulink/Logic and Bit Operations/Detect Change  vinit=boolean(0)  OutDataTypeStr=boolean
  Detect Increase : simulink/Logic and Bit Operations/Detect Increase  vinit=boolean(0)  OutDataTypeStr=boolean
  Equal : RelationalOperator  Operator===  OutDataTypeStr=boolean  RndMeth=Simplest
  Equal1 : RelationalOperator  Operator=~=  OutDataTypeStr=boolean  RndMeth=Simplest
  Equal2 : RelationalOperator  Operator=~=  OutDataTypeStr=boolean  RndMeth=Simplest
  Equal3 : RelationalOperator  Operator===  OutDataTypeStr=boolean  RndMeth=Simplest
  If : If  NumInputs=2  IfExpression=u1 ~=0  ElseIfExpressions=u2 ~= 0
  Maintain : Subsystem  TreatAsAtomicUnit=on
  Merge : Merge  Inputs=3
  OR : Logic  Operator=OR  AllPortsSameDT=off  OutDataTypeStr=boolean
  Reset : Subsystem  TreatAsAtomicUnit=on
  Write : Subsystem  TreatAsAtomicUnit=on
  VSCP_ComboKey2_enum : Outport
  VSCP_Key2Pass_flg : Outport  Port=2
  wires:
  Data Type Conversion/1 -> [VSCP_ComboKey2_enum]  "VTQD_Engineering2_enum"
  [VSCP_ComboKey2_enum] -> Delay2/1
  Delay2/1 -> Maintain/1(Input)
  Equal3/1 -> AND/4
  Delay1/1 -> Equal3/1
  Constant3/1 -> Equal3/2
  [VSCP_ComboKey2_enum] -> Delay1/1
  VSCP_ComboKey1_enum/1 -> [VSCP_ComboKey1_enum]
  OR/1 -> [VSCP_ResetComboKey_flg]  "VSCP_ResetComboKey_flg"
  [VSCP_WriteComboCMD_flg] -> If/2
  [VSCP_ComboKeyCMD_enum] -> Equal1/1
  [VSCP_ComboKeyReset_flg] -> OR/2
  [VSCP_ComboKey1_enum] -> Delay/1
  Equal1/1 -> AND/2
  Constant2/1 -> Equal2/2
  Equal2/1 -> AND/3
  Reset/1(ResetToZero) -> Merge/1
  Merge/1 -> Data Type Conversion/1
  Delay/1 -> Equal2/1
  If/3 -> Maintain/Action
  Constant4/1 -> Equal1/2
  Maintain/1(KeepKey2) -> Merge/3
  Detect Change/1 -> AND/1
  [VSCP_ComboKeyEn_flg] -> Detect Increase/1
  [VSCP_ResetComboKey_flg] -> If/1
  [VSCP_ComboKeyCMD_enum] -> Detect Change/1
  [VSCP_ComboKeyCMD_enum] -> Write/1(Input)
  AND/1 -> [VSCP_WriteComboCMD_flg]  "VSCP_WriteComboCMD_flg"
  Detect Increase/1 -> OR/1
  If/1 -> Reset/Action
  Write/1(WriteCMD) -> Merge/2
  If/2 -> Write/Action
  [VSCP_ComboKey2_enum] -> Equal/1
  Constant1/1 -> Equal/2
  Equal/1 -> [VSCP_Key2Pass_flg]  "VTQD_Engineering2Pass_flg"
  VSCP_ComboKeyCMD_enum/1 -> [VSCP_ComboKeyCMD_enum]
  VSCP_ComboKeyReset_flg/1 -> [VSCP_ComboKeyReset_flg]
  VSCP_ComboKeyEn_flg/1 -> [VSCP_ComboKeyEn_flg]
  [VSCP_ComboKey2_enum] -> VSCP_ComboKey2_enum/1
  [VSCP_Key2Pass_flg] -> VSCP_Key2Pass_flg/1

== system tqdtqr_rebuild_V3/Input_Convert/Signal function/combo key/Combo Key Detection/Engineering Mode/Key3 ==
  VSCP_ComboKeyCMD_enum : Inport
  VSCP_ComboKeyEn_flg : Inport  Port=2
  VSCP_ComboKeyReset_flg : Inport  Port=3
  VSCP_ComboKey2_enum : Inport  Port=4
  AND : Logic  Inputs=4  AllPortsSameDT=off  OutDataTypeStr=boolean
  Constant1 : Constant  Value=KTQD_Engineering3_enum
  Constant2 : Constant  Value=ENUM_COMBOKEY_NONE
  Constant3 : Constant  Value=ENUM_COMBOKEY_NONE
  Constant4 : Constant  Value=ENUM_COMBOKEY_NONE
  Data Type Conversion : DataTypeConversion  OutDataTypeStr=uint8
  Delay : Delay  DelayLength=1  InitialCondition=uint8(0)
      settings: AttributesFormatString=%<InitialCondition>
  Delay1 : Delay  DelayLength=1  InitialCondition=uint8(0)
      settings: AttributesFormatString=%<InitialCondition>
  Delay2 : Delay  DelayLength=1  InitialCondition=uint8(0)
      settings: AttributesFormatString=%<InitialCondition>
  Detect Change : simulink/Logic and Bit Operations/Detect Change  vinit=boolean(0)  OutDataTypeStr=boolean
  Detect Increase : simulink/Logic and Bit Operations/Detect Increase  vinit=boolean(0)  OutDataTypeStr=boolean
  Equal : RelationalOperator  Operator===  OutDataTypeStr=boolean  RndMeth=Simplest
  Equal1 : RelationalOperator  Operator=~=  OutDataTypeStr=boolean  RndMeth=Simplest
  Equal2 : RelationalOperator  Operator=~=  OutDataTypeStr=boolean  RndMeth=Simplest
  Equal3 : RelationalOperator  Operator===  OutDataTypeStr=boolean  RndMeth=Simplest
  If : If  NumInputs=2  IfExpression=u1 ~=0  ElseIfExpressions=u2 ~= 0
  Maintain : Subsystem  TreatAsAtomicUnit=on
  Merge : Merge  Inputs=3
  OR : Logic  Operator=OR  AllPortsSameDT=off  OutDataTypeStr=boolean
  Reset : Subsystem  TreatAsAtomicUnit=on
  Write : Subsystem  TreatAsAtomicUnit=on
  VSCP_ComboKey3_enum : Outport
  VSCP_Key3Pass_flg : Outport  Port=2
  wires:
  Data Type Conversion/1 -> [VSCP_ComboKey3_enum]  "VTQD_Engineering3_enum"
  [VSCP_ComboKey3_enum] -> Delay2/1
  Delay2/1 -> Maintain/1(Input)
  [VSCP_ComboKey3_enum] -> Delay1/1
  Constant3/1 -> Equal3/2
  Equal3/1 -> AND/4
  Delay1/1 -> Equal3/1
  [VSCP_Key3Pass_flg] -> VSCP_Key3Pass_flg/1
  [VSCP_ComboKey3_enum] -> Equal/1
  [VSCP_ComboKey3_enum] -> VSCP_ComboKey3_enum/1
  VSCP_ComboKeyEn_flg/1 -> [VSCP_ComboKeyEn_flg]
  VSCP_ComboKeyReset_flg/1 -> [VSCP_ComboKeyReset_flg]
  VSCP_ComboKeyCMD_enum/1 -> [VSCP_ComboKeyCMD_enum]
  Equal/1 -> [VSCP_Key3Pass_flg]  "VTQD_Engineering3Pass_flg"
  Constant1/1 -> Equal/2
  If/2 -> Write/Action
  Write/1(WriteCMD) -> Merge/2
  If/1 -> Reset/Action
  Detect Increase/1 -> OR/1
  AND/1 -> [VSCP_WriteComboCMD_flg]  "VSCP_WriteComboCMD_flg"
  [VSCP_ComboKeyCMD_enum] -> Write/1(Input)
  [VSCP_ComboKeyCMD_enum] -> Detect Change/1
  [VSCP_ResetComboKey_flg] -> If/1
  [VSCP_ComboKeyEn_flg] -> Detect Increase/1
  Detect Change/1 -> AND/1
  Maintain/1(KeepKey3) -> Merge/3
  Constant4/1 -> Equal1/2
  If/3 -> Maintain/Action
  Delay/1 -> Equal2/1
  Merge/1 -> Data Type Conversion/1
  Reset/1(ResetToZero) -> Merge/1
  Equal2/1 -> AND/3
  Constant2/1 -> Equal2/2
  Equal1/1 -> AND/2
  [VSCP_ComboKey2_enum] -> Delay/1
  [VSCP_ComboKeyReset_flg] -> OR/2
  [VSCP_ComboKeyCMD_enum] -> Equal1/1
  [VSCP_WriteComboCMD_flg] -> If/2
  OR/1 -> [VSCP_ResetComboKey_flg]  "VSCP_ResetComboKey_flg"
  VSCP_ComboKey2_enum/1 -> [VSCP_ComboKey2_enum]

== system tqdtqr_rebuild_V3/Input_Convert/Signal function/combo key/Combo Key Detection/Engineering Mode/Key4 ==
  VSCP_ComboKeyCMD_enum : Inport
  VSCP_ComboKeyEn_flg : Inport  Port=2
  VSCP_ComboKeyReset_flg : Inport  Port=3
  VSCP_ComboKey3_enum : Inport  Port=4
  AND : Logic  Inputs=4  AllPortsSameDT=off  OutDataTypeStr=boolean
  Constant1 : Constant  Value=KTQD_Engineering4_enum
  Constant2 : Constant  Value=ENUM_COMBOKEY_NONE
  Constant3 : Constant  Value=ENUM_COMBOKEY_NONE
  Constant4 : Constant  Value=ENUM_COMBOKEY_NONE
  Data Type Conversion : DataTypeConversion  OutDataTypeStr=uint8
  Delay : Delay  DelayLength=1  InitialCondition=uint8(0)
      settings: AttributesFormatString=%<InitialCondition>
  Delay1 : Delay  DelayLength=1  InitialCondition=uint8(0)
      settings: AttributesFormatString=%<InitialCondition>
  Delay2 : Delay  DelayLength=1  InitialCondition=uint8(0)
      settings: AttributesFormatString=%<InitialCondition>
  Detect Change : simulink/Logic and Bit Operations/Detect Change  vinit=boolean(0)  OutDataTypeStr=boolean
  Detect Increase : simulink/Logic and Bit Operations/Detect Increase  vinit=boolean(0)  OutDataTypeStr=boolean
  Equal : RelationalOperator  Operator===  OutDataTypeStr=boolean  RndMeth=Simplest
  Equal1 : RelationalOperator  Operator=~=  OutDataTypeStr=boolean  RndMeth=Simplest
  Equal2 : RelationalOperator  Operator=~=  OutDataTypeStr=boolean  RndMeth=Simplest
  Equal3 : RelationalOperator  Operator===  OutDataTypeStr=boolean  RndMeth=Simplest
  If : If  NumInputs=2  IfExpression=u1 ~=0  ElseIfExpressions=u2 ~= 0
  Maintain : Subsystem  TreatAsAtomicUnit=on
  Merge : Merge  Inputs=3
  OR : Logic  Operator=OR  AllPortsSameDT=off  OutDataTypeStr=boolean
  Reset : Subsystem  TreatAsAtomicUnit=on
  Write : Subsystem  TreatAsAtomicUnit=on
  VSCP_ComboKey4_enum : Outport
  VSCP_Key4Pass_flg : Outport  Port=2
  wires:
  Data Type Conversion/1 -> [VSCP_ComboKey4_enum]  "VTQD_Engineering4_enum"
  Delay2/1 -> Maintain/1(Input)
  [VSCP_ComboKey4_enum] -> Delay2/1
  [VSCP_ComboKey4_enum] -> VSCP_ComboKey4_enum/1
  [VSCP_Key4Pass_flg] -> VSCP_Key4Pass_flg/1
  Equal3/1 -> AND/4
  Delay1/1 -> Equal3/1
  Constant3/1 -> Equal3/2
  [VSCP_ComboKey4_enum] -> Delay1/1
  VSCP_ComboKey3_enum/1 -> [VSCP_ComboKey3_enum]
  OR/1 -> [VSCP_ResetComboKey_flg]  "VSCP_ResetComboKey_flg"
  [VSCP_WriteComboCMD_flg] -> If/2
  [VSCP_ComboKeyCMD_enum] -> Equal1/1
  [VSCP_ComboKeyReset_flg] -> OR/2
  [VSCP_ComboKey3_enum] -> Delay/1
  Equal1/1 -> AND/2
  Constant2/1 -> Equal2/2
  Equal2/1 -> AND/3
  Reset/1(ResetToZero) -> Merge/1
  Merge/1 -> Data Type Conversion/1
  Delay/1 -> Equal2/1
  If/3 -> Maintain/Action
  Constant4/1 -> Equal1/2
  Maintain/1(KeepKey4) -> Merge/3
  Detect Change/1 -> AND/1
  [VSCP_ComboKeyEn_flg] -> Detect Increase/1
  [VSCP_ResetComboKey_flg] -> If/1
  [VSCP_ComboKeyCMD_enum] -> Detect Change/1
  [VSCP_ComboKeyCMD_enum] -> Write/1(Input)
  AND/1 -> [VSCP_WriteComboCMD_flg]  "VSCP_WriteComboCMD_flg"
  Detect Increase/1 -> OR/1
  If/1 -> Reset/Action
  Write/1(WriteCMD) -> Merge/2
  If/2 -> Write/Action
  Constant1/1 -> Equal/2
  Equal/1 -> [VSCP_Key4Pass_flg]  "VTQD_Engineering4Pass_flg"
  VSCP_ComboKeyCMD_enum/1 -> [VSCP_ComboKeyCMD_enum]
  VSCP_ComboKeyReset_flg/1 -> [VSCP_ComboKeyReset_flg]
  VSCP_ComboKeyEn_flg/1 -> [VSCP_ComboKeyEn_flg]
  [VSCP_ComboKey4_enum] -> Equal/1

== system tqdtqr_rebuild_V3/Input_Convert/Signal function/combo key/Combo Key Detection/Engineering Mode/Key5 ==
  VSCP_ComboKeyCMD_enum : Inport
  VSCP_ComboKeyEn_flg : Inport  Port=2
  VSCP_ComboKeyReset_flg : Inport  Port=3
  VSCP_ComboKey4_enum : Inport  Port=4
  AND : Logic  Inputs=4  AllPortsSameDT=off  OutDataTypeStr=boolean
  Constant1 : Constant  Value=KTQD_Engineering5_enum
  Constant2 : Constant  Value=ENUM_COMBOKEY_NONE
  Constant3 : Constant  Value=ENUM_COMBOKEY_NONE
  Constant4 : Constant  Value=ENUM_COMBOKEY_NONE
  Data Type Conversion : DataTypeConversion  OutDataTypeStr=uint8
  Delay : Delay  DelayLength=1  InitialCondition=uint8(0)
      settings: AttributesFormatString=%<InitialCondition>
  Delay1 : Delay  DelayLength=1  InitialCondition=uint8(0)
      settings: AttributesFormatString=%<InitialCondition>
  Delay2 : Delay  DelayLength=1  InitialCondition=uint8(0)
      settings: AttributesFormatString=%<InitialCondition>
  Detect Change : simulink/Logic and Bit Operations/Detect Change  vinit=boolean(0)  OutDataTypeStr=boolean
  Detect Increase : simulink/Logic and Bit Operations/Detect Increase  vinit=boolean(0)  OutDataTypeStr=boolean
  Equal : RelationalOperator  Operator===  OutDataTypeStr=boolean  RndMeth=Simplest
  Equal1 : RelationalOperator  Operator=~=  OutDataTypeStr=boolean  RndMeth=Simplest
  Equal2 : RelationalOperator  Operator=~=  OutDataTypeStr=boolean  RndMeth=Simplest
  Equal3 : RelationalOperator  Operator===  OutDataTypeStr=boolean  RndMeth=Simplest
  If : If  NumInputs=2  IfExpression=u1 ~=0  ElseIfExpressions=u2 ~= 0
  Maintain : Subsystem  TreatAsAtomicUnit=on
  Merge : Merge  Inputs=3
  OR : Logic  Operator=OR  AllPortsSameDT=off  OutDataTypeStr=boolean
  Reset : Subsystem  TreatAsAtomicUnit=on
  Write : Subsystem  TreatAsAtomicUnit=on
  VSCP_ComboKey5_enum : Outport
  VSCP_Key5Pass_flg : Outport  Port=2
  wires:
  Data Type Conversion/1 -> [VSCP_ComboKey5_enum]  "VTQD_Engineering5_enum"
  Delay2/1 -> Maintain/1(Input)
  [VSCP_ComboKey5_enum] -> Delay2/1
  [VSCP_ComboKey5_enum] -> VSCP_ComboKey5_enum/1
  [VSCP_ComboKey5_enum] -> Equal/1
  VSCP_ComboKeyEn_flg/1 -> [VSCP_ComboKeyEn_flg]
  VSCP_ComboKeyReset_flg/1 -> [VSCP_ComboKeyReset_flg]
  VSCP_ComboKeyCMD_enum/1 -> [VSCP_ComboKeyCMD_enum]
  Equal/1 -> [VSCP_Key5Pass_flg]  "VTQD_Engineering5Pass_flg"
  Constant1/1 -> Equal/2
  If/2 -> Write/Action
  Write/1(WriteCMD) -> Merge/2
  If/1 -> Reset/Action
  Detect Increase/1 -> OR/1
  AND/1 -> [VSCP_WriteComboCMD_flg]  "VSCP_WriteComboCMD_flg"
  [VSCP_ComboKeyCMD_enum] -> Write/1(Input)
  [VSCP_ComboKeyCMD_enum] -> Detect Change/1
  [VSCP_ResetComboKey_flg] -> If/1
  [VSCP_ComboKeyEn_flg] -> Detect Increase/1
  Detect Change/1 -> AND/1
  Maintain/1(KeepKey5) -> Merge/3
  Constant4/1 -> Equal1/2
  If/3 -> Maintain/Action
  Delay/1 -> Equal2/1
  Merge/1 -> Data Type Conversion/1
  Reset/1(ResetToZero) -> Merge/1
  Equal2/1 -> AND/3
  Constant2/1 -> Equal2/2
  Equal1/1 -> AND/2
  [VSCP_ComboKey4_enum] -> Delay/1
  [VSCP_ComboKeyReset_flg] -> OR/2
  [VSCP_ComboKeyCMD_enum] -> Equal1/1
  [VSCP_WriteComboCMD_flg] -> If/2
  OR/1 -> [VSCP_ResetComboKey_flg]  "VSCP_ResetComboKey_flg"
  VSCP_ComboKey4_enum/1 -> [VSCP_ComboKey4_enum]
  [VSCP_ComboKey5_enum] -> Delay1/1
  Constant3/1 -> Equal3/2
  Delay1/1 -> Equal3/1
  Equal3/1 -> AND/4
  [VSCP_Key5Pass_flg] -> VSCP_Key5Pass_flg/1

== system tqdtqr_rebuild_V3/Input_Convert/Signal function/combo key/Combo Key Detection/Engineering Mode/Key6 ==
  VSCP_ComboKeyCMD_enum : Inport
  VSCP_ComboKeyEn_flg : Inport  Port=2
  VSCP_ComboKeyReset_flg : Inport  Port=3
  VSCP_ComboKey5_enum : Inport  Port=4
  AND : Logic  Inputs=4  AllPortsSameDT=off  OutDataTypeStr=boolean
  Constant1 : Constant  Value=KTQD_Engineering6_enum
  Constant2 : Constant  Value=ENUM_COMBOKEY_NONE
  Constant3 : Constant  Value=ENUM_COMBOKEY_NONE
  Constant4 : Constant  Value=ENUM_COMBOKEY_NONE
  Data Type Conversion : DataTypeConversion  OutDataTypeStr=uint8
  Delay : Delay  DelayLength=1  InitialCondition=uint8(0)
      settings: AttributesFormatString=%<InitialCondition>
  Delay1 : Delay  DelayLength=1  InitialCondition=uint8(0)
      settings: AttributesFormatString=%<InitialCondition>
  Delay2 : Delay  DelayLength=1  InitialCondition=uint8(0)
      settings: AttributesFormatString=%<InitialCondition>
  Detect Change : simulink/Logic and Bit Operations/Detect Change  vinit=boolean(0)  OutDataTypeStr=boolean
  Detect Increase : simulink/Logic and Bit Operations/Detect Increase  vinit=boolean(0)  OutDataTypeStr=boolean
  Equal : RelationalOperator  Operator===  OutDataTypeStr=boolean  RndMeth=Simplest
  Equal1 : RelationalOperator  Operator=~=  OutDataTypeStr=boolean  RndMeth=Simplest
  Equal2 : RelationalOperator  Operator=~=  OutDataTypeStr=boolean  RndMeth=Simplest
  Equal3 : RelationalOperator  Operator===  OutDataTypeStr=boolean  RndMeth=Simplest
  If : If  NumInputs=2  IfExpression=u1 ~=0  ElseIfExpressions=u2 ~= 0
  Maintain : Subsystem  TreatAsAtomicUnit=on
  Merge : Merge  Inputs=3
  OR : Logic  Operator=OR  AllPortsSameDT=off  OutDataTypeStr=boolean
  Reset : Subsystem  TreatAsAtomicUnit=on
  Write : Subsystem  TreatAsAtomicUnit=on
  VSCP_ComboKey6_enum : Outport
  VSCP_Key6Pass_flg : Outport  Port=2
  wires:
  Data Type Conversion/1 -> [VSCP_ComboKey6_enum]  "VTQD_Engineering6_enum"
  [VSCP_ComboKey6_enum] -> Delay2/1
  Delay2/1 -> Maintain/1(Input)
  [VSCP_Key6Pass_flg] -> VSCP_Key6Pass_flg/1
  Equal3/1 -> AND/4
  Delay1/1 -> Equal3/1
  Constant3/1 -> Equal3/2
  [VSCP_ComboKey6_enum] -> Delay1/1
  VSCP_ComboKey5_enum/1 -> [VSCP_ComboKey5_enum]
  OR/1 -> [VSCP_ResetComboKey_flg]  "VSCP_ResetComboKey_flg"
  [VSCP_WriteComboCMD_flg] -> If/2
  [VSCP_ComboKeyCMD_enum] -> Equal1/1
  [VSCP_ComboKeyReset_flg] -> OR/2
  [VSCP_ComboKey5_enum] -> Delay/1
  Equal1/1 -> AND/2
  Constant2/1 -> Equal2/2
  Equal2/1 -> AND/3
  Reset/1(ResetToZero) -> Merge/1
  Merge/1 -> Data Type Conversion/1
  Delay/1 -> Equal2/1
  If/3 -> Maintain/Action
  Constant4/1 -> Equal1/2
  Maintain/1(KeepKey6) -> Merge/3
  Detect Change/1 -> AND/1
  [VSCP_ComboKeyEn_flg] -> Detect Increase/1
  [VSCP_ResetComboKey_flg] -> If/1
  [VSCP_ComboKeyCMD_enum] -> Detect Change/1
  [VSCP_ComboKeyCMD_enum] -> Write/1(Input)
  AND/1 -> [VSCP_WriteComboCMD_flg]  "VSCP_WriteComboCMD_flg"
  Detect Increase/1 -> OR/1
  If/1 -> Reset/Action
  Write/1(WriteCMD) -> Merge/2
  If/2 -> Write/Action
  Constant1/1 -> Equal/2
  Equal/1 -> [VSCP_Key6Pass_flg]  "VTQD_Engineering6Pass_flg"
  VSCP_ComboKeyCMD_enum/1 -> [VSCP_ComboKeyCMD_enum]
  VSCP_ComboKeyReset_flg/1 -> [VSCP_ComboKeyReset_flg]
  VSCP_ComboKeyEn_flg/1 -> [VSCP_ComboKeyEn_flg]
  [VSCP_ComboKey6_enum] -> Equal/1
  [VSCP_ComboKey6_enum] -> VSCP_ComboKey6_enum/1
